simulink model "mbd_example_ic"  (R2022b)
settings: Solver=FixedStepDiscrete  StartTime=0.0  StopTime=10.0  RelTol=1e-3  EnableMultiTasking=on
PostLoadFcn:
  | run([bdroot '_init']);
InitFcn:
  | checkModelFolder(true); % Optional
  | run([bdroot '_init']);
model workspace (MAT data in the model file):
  MBDPortal_MaskInitParam = 0
  MBDPortal_MaskInitSignal = 0
  MBDSnap_MaskInitSignal = 0
values from neighbouring files (symbols this model uses):
  MBDDiag_Comm_Module = [2 3]    [mbd_example_ic_init.m]
  MBDDiag_Comm_Speed = [921600 921600]    [mbd_example_ic_init.m]
  T_s_LED1 = 1/LED1_Hz    (= 0.5)    [mbd_example_ic_init.m]
  T_s_LED2 = 1/LED2_Hz    (= 1)    [mbd_example_ic_init.m]
libraries: MbdLib_PortalDiag x18, MbdLib_Digital x10, MbdLib_Uart x6, MbdLib_Pwm x6, MbdLib_Timer x6, MbdLib_Ic x4, MbdLib_SnapDiag x2, MbdLib_Required x1
settings Model: Creator=KenYoshioka  LastModifiedBy=KenYoshioka
settings SolverCC: AutoInsertRateTranBlk=on
settings OptimizationCC: DefaultParameterBehavior=Inlined  DefaultUnderspecifiedDataType=single  EnhancedBackFolding=on  BooleansAsBitfields=on  PassReuseOutputArgsAs=Individual arguments  ZeroExternalMemoryAtStartup=off  ZeroInternalMemoryAtStartup=off  OptimizeBlockOrder=speed  DifferentSizesBufferReuse=on  EfficientTunableParamExpr=on
settings DebuggingCC: MultiTaskDSMMsg=none  ParameterTunabilityLossMsg=error
settings HardwareCC: ProdBitPerPointer=32  ProdBitPerSizeT=32  ProdBitPerPtrDiffT=32  ProdLargestAtomicInteger=Long  ProdLargestAtomicFloat=Double  ProdWordSize=32  ProdHWDeviceType=ARM Compatible->ARM Cortex-M
settings ModelReferenceCC: EnableRefExpFcnMdlSchedulingChecks=on  ModelReferenceNumInstancesAllowed=Single
settings SFSimCC: MATLABDynamicMemAlloc=off
settings RTWCC: Description=MBD Embedded Target STM32 Cortex M4 (real-time)  SystemTargetFile=MBD_STM32_stf.tlc  TemplateMakefile=MBD_STM32.tmf  Toolchain=arm-none-eabi - v9.3.1
settings CodeAppCC: ForceParamTrailComments=on  IgnoreCustomStorageClasses=off  MaxIdLength=255  OperatorAnnotations=on  SimulinkDataObjDesc=on  SFDataObjDesc=on  InsertBlockDesc=on
settings STFCustomTargetCC: MultiwordLength=256  IncludeMdlTerminateFcn=off  CombineOutputUpdateFcns=on  CombineSignalStateStructs=on  SuppressErrorStatus=on  ERTCustomFileBanners=on  SupportContinuousTime=off  RemoveResetFunc=on  MATLABClassNameForMDSCustomization=Simulink.SoftwareTarget.ERTCustomization  UseToolchainInfoCompliant=on  SystemTargetFile=MBD_STM32_stf.tlc
settings ERTTargetCC: ParMdlRefBuildCompliant=off  CompOptLevelCompliant=off  ConcurrentExecutionCompliant=off  IncludeMdlTerminateFcn=off  CombineSignalStateStructs=on  SuppressErrorStatus=on  SupportNonInlinedSFcns=on  ModelStepFunctionPrototypeControlCompliant=off  CPPClassGenCompliant=off  ExtModeStaticAllocSize=2000  InlinedParameterPlacement=NonHierarchical  ERTCustomFileTemplate=mbd_lib_interface.tlc  MaxLineWidth=110

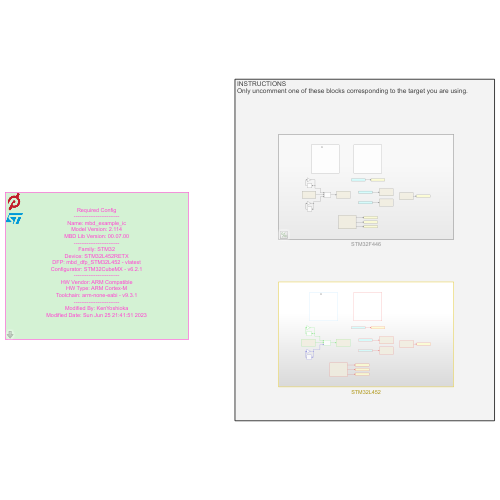
[thumbnail: Simulink's stored preview of the top-level diagram]
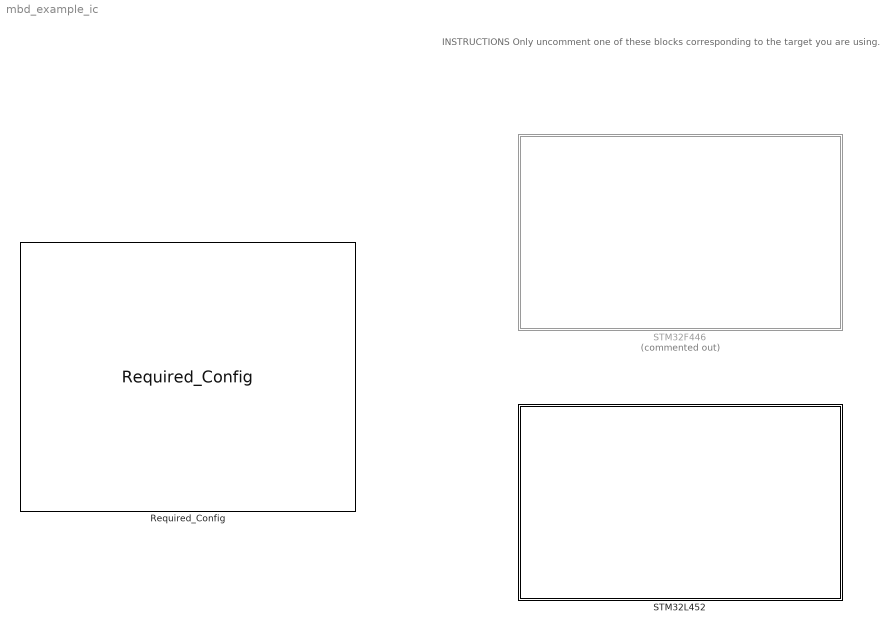
== system mbd_example_ic ==
  note: INSTRUCTIONS
      | Only uncomment one of these blocks corresponding to the target you are using.
  Required_Config : MbdLib_Required/Required_Config  Tag=MBD_Target_Info  Param_update=1
      settings: SourceProductName=Peloton Interface Library
  STM32F446 : Subsystem  Commented=on
  STM32L452 : Subsystem

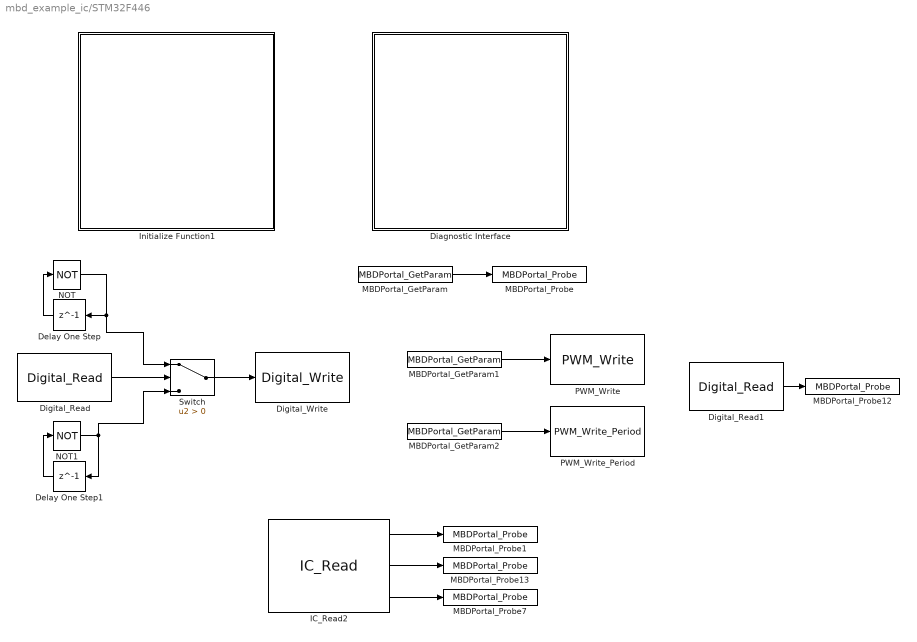
== system mbd_example_ic/STM32F446 ==
  Delay One Step : Delay  DelayLength=1  SampleTime=T_s_LED1
  Delay One Step1 : Delay  DelayLength=1  SampleTime=T_s_LED2
  Diagnostic Interface : Subsystem
  Digital_Read : MbdLib_Digital/Digital_Read  Param_module=C  Param_ch=13  Param_sampleTime=-1  Sim_invert=off  Sim_out=0
      settings: SourceProductName=Peloton Interface Library
  Digital_Read1 : MbdLib_Digital/Digital_Read  Param_module=A  Param_ch=8  Param_sampleTime=-1  Sim_invert=off  Sim_out=0
      settings: SourceProductName=Peloton Interface Library
  Digital_Write : MbdLib_Digital/Digital_Write  Param_module=C  Param_ch=10  Param_sampleTime=-1
      settings: SourceProductName=Peloton Interface Library
  IC_Read2 : MbdLib_Ic/IC_Read  Param_module=1  Param_ch=1  Param_width=byte  Param_length=5  Param_sampleTime=-1
      settings: SourceProductName=Peloton Interface Library
  Initialize Function1 : Subsystem  TreatAsAtomicUnit=on
  MBDPortal_GetParam : MbdLib_PortalDiag/MBDPortal_GetParam  Param_ParamName=Parameter  Param_ParamDefault=0  Param_ParamIndex=0  Param_ParamMax=MBDPortal_ParamNum
      settings: SourceProductName=Peloton Component Library
  MBDPortal_GetParam1 : MbdLib_PortalDiag/MBDPortal_GetParam  Param_ParamName=PWM_duty  Param_ParamDefault=50000000  Param_ParamIndex=0  Param_ParamMax=MBDPortal_ParamNum
      settings: SourceProductName=Peloton Component Library
  MBDPortal_GetParam2 : MbdLib_PortalDiag/MBDPortal_GetParam  Param_ParamName=PWM_period  Param_ParamDefault=100000000  Param_ParamIndex=0  Param_ParamMax=MBDPortal_ParamNum
      settings: SourceProductName=Peloton Component Library
  MBDPortal_Probe : MbdLib_PortalDiag/MBDPortal_Probe  Param_SigNameInherited=on  Param_SigName=Signals  Param_SigIndex=0  Param_SigMax=MBDPortal_SignalNum  Param_SampleTime=MBDPortal_CommonSampleRate
      settings: SourceProductName=Peloton Component Library
  MBDPortal_Probe1 : MbdLib_PortalDiag/MBDPortal_Probe  Param_SigNameInherited=on  Param_SigName=IC_data  Param_SigIndex=0  Param_SigMax=MBDPortal_SignalNum  Param_SampleTime=MBDPortal_CommonSampleRate
      settings: SourceProductName=Peloton Component Library
  MBDPortal_Probe12 : MbdLib_PortalDiag/MBDPortal_Probe  Param_SigNameInherited=on  Param_SigName=PWM_in  Param_SigIndex=0  Param_SigMax=MBDPortal_SignalNum  Param_SampleTime=MBDPortal_CommonSampleRate
      settings: SourceProductName=Peloton Component Library
  MBDPortal_Probe13 : MbdLib_PortalDiag/MBDPortal_Probe  Param_SigNameInherited=on  Param_SigName=IC_count  Param_SigIndex=0  Param_SigMax=MBDPortal_SignalNum  Param_SampleTime=MBDPortal_CommonSampleRate
      settings: SourceProductName=Peloton Component Library
  MBDPortal_Probe7 : MbdLib_PortalDiag/MBDPortal_Probe  Param_SigNameInherited=on  Param_SigName=IC_status  Param_SigIndex=0  Param_SigMax=MBDPortal_SignalNum  Param_SampleTime=MBDPortal_CommonSampleRate
      settings: SourceProductName=Peloton Component Library
  NOT : Logic  Operator=NOT  IconShape=distinctive  AllPortsSameDT=off  OutDataTypeStr=boolean
  NOT1 : Logic  Operator=NOT  IconShape=distinctive  AllPortsSameDT=off  OutDataTypeStr=boolean
  PWM_Write : MbdLib_Pwm/PWM_Write  Param_module=2  Param_ch_visible=1  Param_ch=1  Param_sync=off  Param_sampleTime=-1
      settings: SourceProductName=Peloton Interface Library
  PWM_Write_Period : MbdLib_Pwm/PWM_Write_Period  Param_module=2  Param_sampleTime=-1
      settings: SourceProductName=Peloton Interface Library
  Switch : Switch  Criteria=u2 > Threshold  SaturateOnIntegerOverflow=off  InputSameDT=off
  wires:
  MBDPortal_GetParam1/1 -> PWM_Write/1
  MBDPortal_GetParam2/1 -> PWM_Write_Period/1
  Digital_Read1/1 -> MBDPortal_Probe12/1
  Digital_Read/1 -> Switch/2
  NOT/1 -> Switch/1, Delay One Step/1
  MBDPortal_GetParam/1 -> MBDPortal_Probe/1
  Delay One Step1/1 -> NOT1/1
  NOT1/1 -> Switch/3, Delay One Step1/1
  Switch/1 -> Digital_Write/1
  Delay One Step/1 -> NOT/1
  IC_Read2/2 -> MBDPortal_Probe13/1
  IC_Read2/1 -> MBDPortal_Probe1/1
  IC_Read2/3 -> MBDPortal_Probe7/1

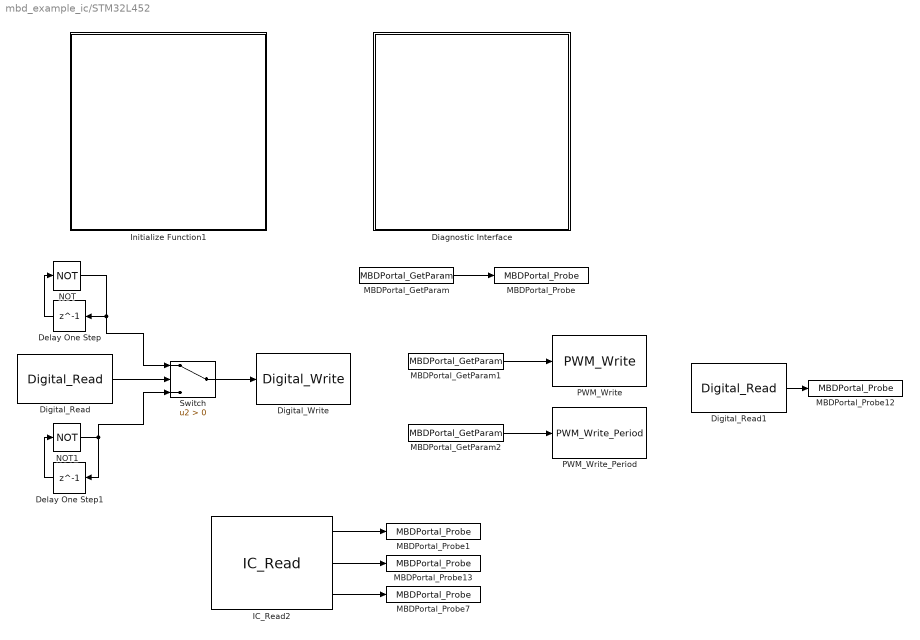
== system mbd_example_ic/STM32L452 ==
  Delay One Step : Delay  DelayLength=1  SampleTime=T_s_LED1
  Delay One Step1 : Delay  DelayLength=1  SampleTime=T_s_LED2
  Diagnostic Interface : Subsystem
  Digital_Read : MbdLib_Digital/Digital_Read  Param_module=C  Param_ch=13  Param_sampleTime=-1  Sim_invert=off  Sim_out=0
      settings: SourceProductName=Peloton Interface Library
  Digital_Read1 : MbdLib_Digital/Digital_Read  Param_module=A  Param_ch=8  Param_sampleTime=-1  Sim_invert=off  Sim_out=0
      settings: SourceProductName=Peloton Interface Library
  Digital_Write : MbdLib_Digital/Digital_Write  Param_module=C  Param_ch=10  Param_sampleTime=-1
      settings: SourceProductName=Peloton Interface Library
  IC_Read2 : MbdLib_Ic/IC_Read  Param_module=1  Param_ch=1  Param_width=byte  Param_length=5  Param_sampleTime=-1
      settings: SourceProductName=Peloton Interface Library
  Initialize Function1 : Subsystem  TreatAsAtomicUnit=on
  MBDPortal_GetParam : MbdLib_PortalDiag/MBDPortal_GetParam  Param_ParamName=Parameter  Param_ParamDefault=0  Param_ParamIndex=0  Param_ParamMax=MBDPortal_ParamNum
      settings: SourceProductName=Peloton Component Library
  MBDPortal_GetParam1 : MbdLib_PortalDiag/MBDPortal_GetParam  Param_ParamName=PWM_duty  Param_ParamDefault=5000  Param_ParamIndex=0  Param_ParamMax=MBDPortal_ParamNum
      settings: SourceProductName=Peloton Component Library
  MBDPortal_GetParam2 : MbdLib_PortalDiag/MBDPortal_GetParam  Param_ParamName=PWM_period  Param_ParamDefault=10000  Param_ParamIndex=0  Param_ParamMax=MBDPortal_ParamNum
      settings: SourceProductName=Peloton Component Library
  MBDPortal_Probe : MbdLib_PortalDiag/MBDPortal_Probe  Param_SigNameInherited=on  Param_SigName=Signals  Param_SigIndex=0  Param_SigMax=MBDPortal_SignalNum  Param_SampleTime=MBDPortal_CommonSampleRate
      settings: SourceProductName=Peloton Component Library
  MBDPortal_Probe1 : MbdLib_PortalDiag/MBDPortal_Probe  Param_SigNameInherited=on  Param_SigName=IC_data  Param_SigIndex=0  Param_SigMax=MBDPortal_SignalNum  Param_SampleTime=MBDPortal_CommonSampleRate
      settings: SourceProductName=Peloton Component Library
  MBDPortal_Probe12 : MbdLib_PortalDiag/MBDPortal_Probe  Param_SigNameInherited=on  Param_SigName=PWM_in  Param_SigIndex=0  Param_SigMax=MBDPortal_SignalNum  Param_SampleTime=MBDPortal_CommonSampleRate
      settings: SourceProductName=Peloton Component Library
  MBDPortal_Probe13 : MbdLib_PortalDiag/MBDPortal_Probe  Param_SigNameInherited=on  Param_SigName=IC_count  Param_SigIndex=0  Param_SigMax=MBDPortal_SignalNum  Param_SampleTime=MBDPortal_CommonSampleRate
      settings: SourceProductName=Peloton Component Library
  MBDPortal_Probe7 : MbdLib_PortalDiag/MBDPortal_Probe  Param_SigNameInherited=on  Param_SigName=IC_status  Param_SigIndex=0  Param_SigMax=MBDPortal_SignalNum  Param_SampleTime=MBDPortal_CommonSampleRate
      settings: SourceProductName=Peloton Component Library
  NOT : Logic  Operator=NOT  IconShape=distinctive  AllPortsSameDT=off  OutDataTypeStr=boolean
  NOT1 : Logic  Operator=NOT  IconShape=distinctive  AllPortsSameDT=off  OutDataTypeStr=boolean
  PWM_Write : MbdLib_Pwm/PWM_Write  Param_module=2  Param_ch_visible=1  Param_ch=1  Param_sync=off  Param_sampleTime=-1
      settings: SourceProductName=Peloton Interface Library
  PWM_Write_Period : MbdLib_Pwm/PWM_Write_Period  Param_module=2  Param_sampleTime=-1
      settings: SourceProductName=Peloton Interface Library
  Switch : Switch  Criteria=u2 > Threshold  SaturateOnIntegerOverflow=off  InputSameDT=off
  wires:
  MBDPortal_GetParam/1 -> MBDPortal_Probe/1
  Delay One Step/1 -> NOT/1
  Digital_Read/1 -> Switch/2
  Delay One Step1/1 -> NOT1/1
  NOT1/1 -> Switch/3, Delay One Step1/1
  Switch/1 -> Digital_Write/1
  NOT/1 -> Switch/1, Delay One Step/1
  MBDPortal_GetParam1/1 -> PWM_Write/1
  MBDPortal_GetParam2/1 -> PWM_Write_Period/1
  Digital_Read1/1 -> MBDPortal_Probe12/1
  IC_Read2/3 -> MBDPortal_Probe7/1
  IC_Read2/2 -> MBDPortal_Probe13/1
  IC_Read2/1 -> MBDPortal_Probe1/1

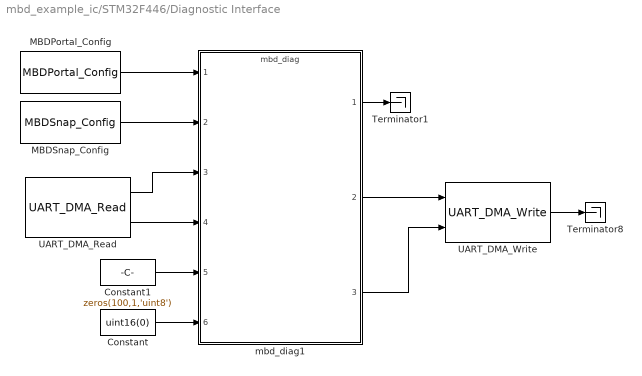
== system mbd_example_ic/STM32F446/Diagnostic Interface ==
  Constant : Constant  Value=uint16(0)
  Constant1 : Constant  Value=zeros(100,1,'uint8')
  MBDPortal_Config : MbdLib_PortalDiag/MBDPortal_Config  Param_SigMax=MBDPortal_SignalNum  Param_ParamMax=MBDPortal_ParamNum
      settings: SourceProductName=Peloton Component Library
  MBDSnap_Config : MbdLib_SnapDiag/MBDSnap_Config  Priority=-5000  Param_enableAll=on  Param_SampleTime=T_s_COMM  Param_SigMax=MBDSnap_SignalNum
      settings: SourceProductName=Peloton Component Library
  Terminator1 : Terminator
  Terminator8 : Terminator
  UART_DMA_Read : MbdLib_Uart/UART_DMA_Read  Tag=TAG_UART_DMA  Param_module=MBDDiag_Comm_Module(1)  Param_type=USART  Param_readLim=100  Param_sampleTime=T_s_COMM
      settings: SourceProductName=Peloton Interface Library
  UART_DMA_Write : MbdLib_Uart/UART_DMA_Write  Param_module=2  Param_type=USART  Param_sampleTime=-1  Sim_status=0
      settings: SourceProductName=Peloton Interface Library
  mbd_diag1 : ModelReference  ModelNameDialog=mbd_diag.slx  SimulationMode=Normal  ModelReferenceVersion=2.247  SimulationMode=Normal
  wires:
  UART_DMA_Read/1 -> mbd_diag1/3
  UART_DMA_Write/1 -> Terminator8/1
  mbd_diag1/1 -> Terminator1/1
  MBDPortal_Config/1 -> mbd_diag1/1
  mbd_diag1/3 -> UART_DMA_Write/2
  MBDSnap_Config/1 -> mbd_diag1/2
  mbd_diag1/2 -> UART_DMA_Write/1
  UART_DMA_Read/2 -> mbd_diag1/4
  Constant1/1 -> mbd_diag1/5
  Constant/1 -> mbd_diag1/6

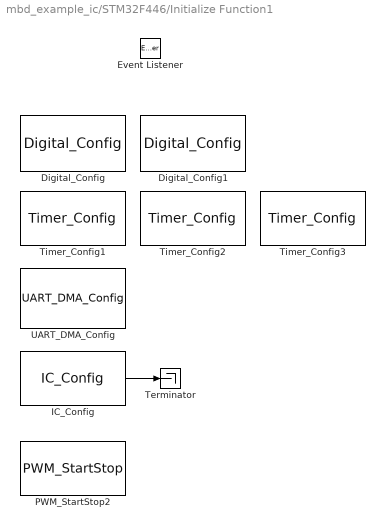
== system mbd_example_ic/STM32F446/Initialize Function1 ==
  Digital_Config : MbdLib_Digital/Digital_Config  Priority=30  Param_module=C  Param_ch=10  Param_dir=output  Param_pupd=none  Param_default=low  Param_mode=none  Param_drive=low  Param_speed=high  Param_priority=30  Param_sampleTime=-1
      settings: AttributesFormatString=priority=%<priority>  SourceProductName=Peloton Interface Library
  Digital_Config1 : MbdLib_Digital/Digital_Config  Priority=30  Param_module=C  Param_ch=13  Param_dir=input  Param_pupd=pullup  Param_default=low  Param_mode=none  Param_drive=low  Param_speed=high  Param_priority=30  Param_sampleTime=-1
      settings: AttributesFormatString=priority=%<priority>  SourceProductName=Peloton Interface Library
  Event Listener : EventListener  DisableCoverage=on  EventName=reset
  IC_Config : MbdLib_Ic/IC_Config  Priority=120  Param_module=1  Param_ch=1  Param_width=halfword  Param_length=5  Param_priority=120  Param_sampleTime=-1
      settings: AttributesFormatString=priority=%<priority>  SourceProductName=Peloton Interface Library
  PWM_StartStop2 : MbdLib_Pwm/PWM_StartStop  Priority=130  Param_module=2  Param_ch=1  Param_action=Start  Param_priority=130  Param_sampleTime=-1
      settings: AttributesFormatString=priority=%<priority>  SourceProductName=Peloton Interface Library
  Terminator : Terminator
  Timer_Config1 : MbdLib_Timer/Timer_Config  Priority=100  Param_update=1  Param_module=1  Param_step=-1  Param_period=0  Param_divider=0  Param_step0=0  Param_clksrc0=0  Param_period0=Comm_period_cycles  Param_divider0=Comm_clock_divider  Param_step1=-1  Param_clksrc1=0  Param_period1=0  Param_divider1=0  Param_step2=-1  Param_clksrc2=0  Param_period2=0  Param_divider2=0  Param_priority=100  Param_sampleTime=-1
      settings: AttributesFormatString=priority=%<priority>  SourceProductName=Peloton Interface Library
  Timer_Config2 : MbdLib_Timer/Timer_Config  Priority=101  Param_update=1  Param_module=6  Param_step=-1  Param_period=0  Param_divider=0  Param_step0=1  Param_clksrc0=0  Param_period0=LED1_period_cycles  Param_divider0=LED1_clock_divider  Param_step1=-1  Param_clksrc1=0  Param_period1=0  Param_divider1=0  Param_step2=-1  Param_clksrc2=0  Param_period2=0  Param_divider2=0  Param_priority=101  Param_sampleTime=-1
      settings: AttributesFormatString=priority=%<priority>  SourceProductName=Peloton Interface Library
  Timer_Config3 : MbdLib_Timer/Timer_Config  Priority=102  Param_update=1  Param_module=7  Param_step=-1  Param_period=0  Param_divider=0  Param_step0=2  Param_clksrc0=0  Param_period0=LED2_period_cycles  Param_divider0=LED2_clock_divider  Param_step1=-1  Param_clksrc1=0  Param_period1=0  Param_divider1=0  Param_step2=-1  Param_clksrc2=0  Param_period2=0  Param_divider2=0  Param_priority=102  Param_sampleTime=-1
      settings: AttributesFormatString=priority=%<priority>  SourceProductName=Peloton Interface Library
  UART_DMA_Config : MbdLib_Uart/UART_DMA_Config  Priority=110  Param_module=MBDDiag_Comm_Module(1)  Param_type=USART  Param_speed=MBDDiag_Comm_Speed(1)  Param_dataBits=8  Param_stopBits=1  Param_parity=None  Param_priority=110  Param_sampleTime=-1
      settings: AttributesFormatString=priority=%<priority>  SourceProductName=Peloton Interface Library
  wires:
  IC_Config/1 -> Terminator/1

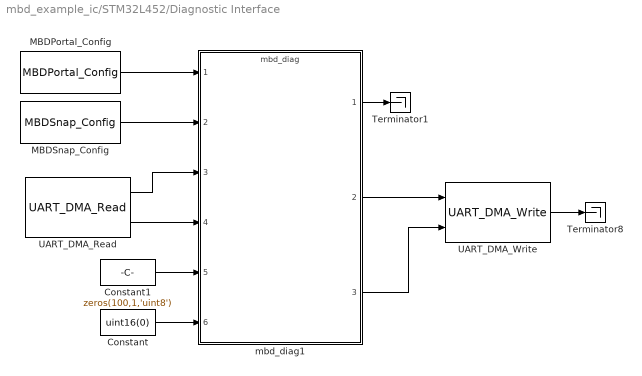
== system mbd_example_ic/STM32L452/Diagnostic Interface ==
  Constant : Constant  Value=uint16(0)
  Constant1 : Constant  Value=zeros(100,1,'uint8')
  MBDPortal_Config : MbdLib_PortalDiag/MBDPortal_Config  Param_SigMax=MBDPortal_SignalNum  Param_ParamMax=MBDPortal_ParamNum
      settings: SourceProductName=Peloton Component Library
  MBDSnap_Config : MbdLib_SnapDiag/MBDSnap_Config  Priority=-5000  Param_enableAll=on  Param_SampleTime=T_s_COMM  Param_SigMax=MBDSnap_SignalNum
      settings: SourceProductName=Peloton Component Library
  Terminator1 : Terminator
  Terminator8 : Terminator
  UART_DMA_Read : MbdLib_Uart/UART_DMA_Read  Tag=TAG_UART_DMA  Param_module=MBDDiag_Comm_Module(1)  Param_type=USART  Param_readLim=100  Param_sampleTime=T_s_COMM
      settings: SourceProductName=Peloton Interface Library
  UART_DMA_Write : MbdLib_Uart/UART_DMA_Write  Param_module=2  Param_type=USART  Param_sampleTime=-1  Sim_status=0
      settings: SourceProductName=Peloton Interface Library
  mbd_diag1 : ModelReference  ModelNameDialog=mbd_diag.slx  SimulationMode=Normal  ModelReferenceVersion=2.247  SimulationMode=Normal
  wires:
  UART_DMA_Read/1 -> mbd_diag1/3
  UART_DMA_Write/1 -> Terminator8/1
  mbd_diag1/1 -> Terminator1/1
  MBDPortal_Config/1 -> mbd_diag1/1
  mbd_diag1/3 -> UART_DMA_Write/2
  MBDSnap_Config/1 -> mbd_diag1/2
  mbd_diag1/2 -> UART_DMA_Write/1
  UART_DMA_Read/2 -> mbd_diag1/4
  Constant1/1 -> mbd_diag1/5
  Constant/1 -> mbd_diag1/6

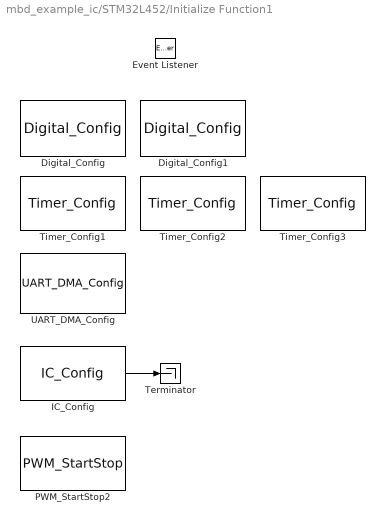
== system mbd_example_ic/STM32L452/Initialize Function1 ==
  Digital_Config : MbdLib_Digital/Digital_Config  Priority=30  Param_module=C  Param_ch=10  Param_dir=output  Param_pupd=none  Param_default=low  Param_mode=none  Param_drive=low  Param_speed=high  Param_priority=30  Param_sampleTime=-1
      settings: AttributesFormatString=priority=%<priority>  SourceProductName=Peloton Interface Library
  Digital_Config1 : MbdLib_Digital/Digital_Config  Priority=30  Param_module=C  Param_ch=13  Param_dir=input  Param_pupd=pullup  Param_default=low  Param_mode=none  Param_drive=low  Param_speed=high  Param_priority=30  Param_sampleTime=-1
      settings: AttributesFormatString=priority=%<priority>  SourceProductName=Peloton Interface Library
  Event Listener : EventListener  DisableCoverage=on  EventName=reset
  IC_Config : MbdLib_Ic/IC_Config  Priority=120  Param_module=1  Param_ch=1  Param_width=halfword  Param_length=5  Param_priority=120  Param_sampleTime=-1
      settings: AttributesFormatString=priority=%<priority>  SourceProductName=Peloton Interface Library
  PWM_StartStop2 : MbdLib_Pwm/PWM_StartStop  Priority=130  Param_module=2  Param_ch=1  Param_action=Start  Param_priority=130  Param_sampleTime=-1
      settings: AttributesFormatString=priority=%<priority>  SourceProductName=Peloton Interface Library
  Terminator : Terminator
  Timer_Config1 : MbdLib_Timer/Timer_Config  Priority=100  Param_update=1  Param_module=6  Param_step=-1  Param_period=0  Param_divider=0  Param_step0=0  Param_clksrc0=0  Param_period0=Comm_period_cycles  Param_divider0=Comm_clock_divider  Param_step1=-1  Param_clksrc1=0  Param_period1=0  Param_divider1=0  Param_step2=-1  Param_clksrc2=0  Param_period2=0  Param_divider2=0  Param_priority=100  Param_sampleTime=-1
      settings: AttributesFormatString=priority=%<priority>  SourceProductName=Peloton Interface Library
  Timer_Config2 : MbdLib_Timer/Timer_Config  Priority=101  Param_update=1  Param_module=15  Param_step=-1  Param_period=0  Param_divider=0  Param_step0=1  Param_clksrc0=0  Param_period0=LED1_period_cycles  Param_divider0=LED1_clock_divider  Param_step1=-1  Param_clksrc1=0  Param_period1=0  Param_divider1=0  Param_step2=-1  Param_clksrc2=0  Param_period2=0  Param_divider2=0  Param_priority=101  Param_sampleTime=-1
      settings: AttributesFormatString=priority=%<priority>  SourceProductName=Peloton Interface Library
  Timer_Config3 : MbdLib_Timer/Timer_Config  Priority=102  Param_update=1  Param_module=16  Param_step=-1  Param_period=0  Param_divider=0  Param_step0=2  Param_clksrc0=0  Param_period0=LED2_period_cycles  Param_divider0=LED2_clock_divider  Param_step1=-1  Param_clksrc1=0  Param_period1=0  Param_divider1=0  Param_step2=-1  Param_clksrc2=0  Param_period2=0  Param_divider2=0  Param_priority=102  Param_sampleTime=-1
      settings: AttributesFormatString=priority=%<priority>  SourceProductName=Peloton Interface Library
  UART_DMA_Config : MbdLib_Uart/UART_DMA_Config  Priority=110  Param_module=MBDDiag_Comm_Module(1)  Param_type=USART  Param_speed=MBDDiag_Comm_Speed(1)  Param_dataBits=8  Param_stopBits=1  Param_parity=None  Param_priority=110  Param_sampleTime=-1
      settings: AttributesFormatString=priority=%<priority>  SourceProductName=Peloton Interface Library
  wires:
  IC_Config/1 -> Terminator/1
